simulink model "plotter_plant"  (R2024b)
settings: Solver=VariableStepAuto  StartTime=0.0  StopTime=10.0  RelTol=1e-3
values from neighbouring files (symbols this model uses):
  MOT_B = 0.001    [init_plotter_data.m]
  MOT_J = 0.01    [init_plotter_data.m]
  MOT_K = 0.1    [init_plotter_data.m]
  MOT_L = 0.5    [init_plotter_data.m]
  MOT_R = 2.0    (= 2)    [init_plotter_data.m]
settings Model: Creator=Niels  LastModifiedBy=Niels

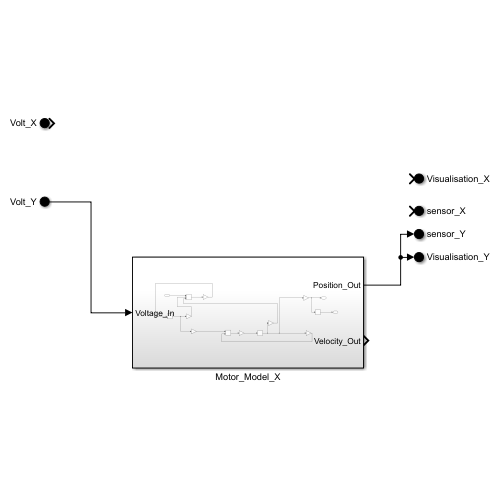
[thumbnail: Simulink's stored preview of the top-level diagram]
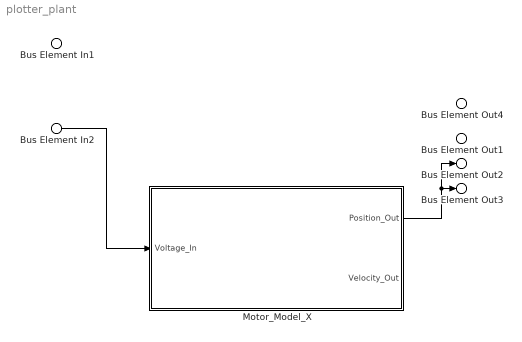
== system plotter_plant ==
  Bus Element In2 : Inport  PortName=Volt_Y
  Bus Element In1 : Inport  Port=2  PortName=Volt_X
  Motor_Model_X : Subsystem
  Bus Element Out1 : Outport  PortName=sensor_X
  Bus Element Out2 : Outport  Port=2  PortName=sensor_Y
  Bus Element Out3 : Outport  Port=3  PortName=Visualisation_Y
  Bus Element Out4 : Outport  Port=4  PortName=Visualisation_X
  wires:
  Bus Element In2/1 -> Motor_Model_X/1(Voltage_In)
  Motor_Model_X/1(Position_Out) -> Bus Element Out2/1, Bus Element Out3/1

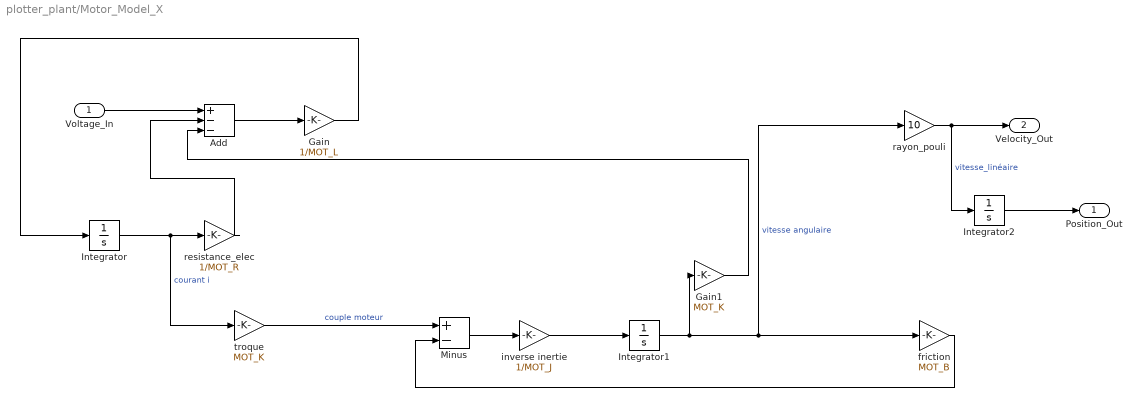
== system plotter_plant/Motor_Model_X ==
  Voltage_In : Inport
  Add : Sum  Inputs=+--
  Gain : Gain  Gain=1/MOT_L
  Gain1 : Gain  Gain=MOT_K
  Integrator : Integrator
  Integrator1 : Integrator
  Integrator2 : Integrator
  Minus : Sum  Inputs=+-
  friction : Gain  Gain=MOT_B
  inverse inertie : Gain  Gain=1/MOT_J
  rayon_pouli : Gain  Gain=10
  resistance_elec : Gain  Gain=1/MOT_R
  troque : Gain  Gain=MOT_K
  Position_Out : Outport
  Velocity_Out : Outport  Port=2
  wires:
  Voltage_In/1 -> Add/1
  Add/1 -> Gain/1
  Integrator/1 -> troque/1, resistance_elec/1  "courant i"
  troque/1 -> Minus/1  "couple moteur"
  Minus/1 -> inverse inertie/1
  inverse inertie/1 -> Integrator1/1
  Integrator1/1 -> Gain1/1, rayon_pouli/1, friction/1  "vitesse angulaire"
  friction/1 -> Minus/2
  Gain/1 -> Integrator/1
  resistance_elec/1 -> Add/2
  Gain1/1 -> Add/3
  rayon_pouli/1 -> Integrator2/1, Velocity_Out/1  "vitesse_linéaire"
  Integrator2/1 -> Position_Out/1
